simulink model "main_model"  (R2019b)
settings: Solver=FixedStepAuto  StartTime=0.0  StopTime=60.0  FixedStep=0.01  MaxStep=0.01  RelTol=1e-3
values from neighbouring files (symbols this model uses):
  data_array_1 = audioread('Model_Data/Microphone_Data/data_array_1/capture.wav')    [set_workspace_parameters.m]
  data_array_2 = audioread('Model_Data/Microphone_Data/data_array_2/capture.wav')    [set_workspace_parameters.m]
  data_array_3 = audioread('Model_Data/Microphone_Data/data_array_3/capture.wav')    [set_workspace_parameters.m]
undefined symbols (not defined in the file or in its folder): __PRM__SERIALIZED__DATA__, BF, pos, SubsystemReferenceBlock
settings Model: Creator=toons  LastModifiedBy=toons
settings DataIOCC: ExternalInput=[input1, input2]  ReturnWorkspaceOutputs=off
settings DebuggingCC: ArithmeticOperatorsInVariantConditions=warning
settings SFSimCC: CustomCodeUndefinedFunction=UseInterfaceOnly

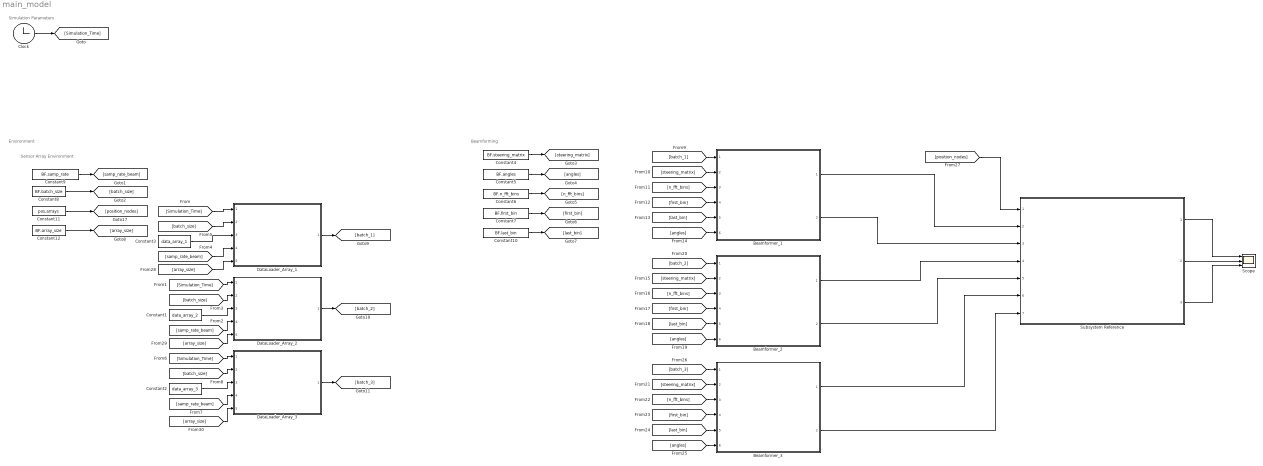
== system main_model ==
  note: Beamforming
  note: Environment
  note: Sensor Array Environment
  note: Simulation Parameters
  Beamformer_1 : Subsystem  BlockKeywords=__PRM__SERIALIZED__DATA__:SubsystemReferenceBlock  ReferencedSubsystem=Beamform_Single_Array
  Beamformer_2 : Subsystem  BlockKeywords=__PRM__SERIALIZED__DATA__:SubsystemReferenceBlock  ReferencedSubsystem=Beamform_Single_Array
  Beamformer_3 : Subsystem  BlockKeywords=__PRM__SERIALIZED__DATA__:SubsystemReferenceBlock  ReferencedSubsystem=Beamform_Single_Array
  Clock : Clock
  Constant1 : Constant  Value=data_array_2  VectorParams1D=off
  Constant10 : Constant  Value=BF.last_bin  VectorParams1D=off
  Constant11 : Constant  Value=pos.arrays  VectorParams1D=off
  Constant12 : Constant  Value=BF.array_size  VectorParams1D=off
  Constant2 : Constant  Value=data_array_3  VectorParams1D=off
  Constant3 : Constant  Value=data_array_1  VectorParams1D=off
  Constant4 : Constant  Value=BF.steering_matrix  VectorParams1D=off
  Constant5 : Constant  Value=BF.angles  VectorParams1D=off
  Constant6 : Constant  Value=BF.n_fft_bins  VectorParams1D=off
  Constant7 : Constant  Value=BF.first_bin  VectorParams1D=off
  Constant8 : Constant  Value=BF.batch_size  VectorParams1D=off
  Constant9 : Constant  Value=BF.samp_rate  VectorParams1D=off
  DataLoader_Array_1 : Subsystem  BlockKeywords=__PRM__SERIALIZED__DATA__:SubsystemReferenceBlock  ReferencedSubsystem=DataLoader_Single_Array
  DataLoader_Array_2 : Subsystem  BlockKeywords=__PRM__SERIALIZED__DATA__:SubsystemReferenceBlock  ReferencedSubsystem=DataLoader_Single_Array
  DataLoader_Array_3 : Subsystem  BlockKeywords=__PRM__SERIALIZED__DATA__:SubsystemReferenceBlock  ReferencedSubsystem=DataLoader_Single_Array
  Scope : Scope  NumInputPorts=3
  Subsystem Reference : Subsystem  BlockKeywords=__PRM__SERIALIZED__DATA__:SubsystemReferenceBlock  ReferencedSubsystem=AnglesToPosition
  wires:
  Clock/1 -> [Simulation_Time]
  Constant3/1 -> DataLoader_Array_1/3
  [Simulation_Time] -> DataLoader_Array_1/1
  Constant9/1 -> [samp_rate_beam]
  [samp_rate_beam] -> DataLoader_Array_1/4
  Constant8/1 -> [batch_size]
  [batch_size] -> DataLoader_Array_1/2
  [batch_size] -> DataLoader_Array_2/2
  Constant1/1 -> DataLoader_Array_2/3
  [Simulation_Time] -> DataLoader_Array_2/1
  [samp_rate_beam] -> DataLoader_Array_2/4
  Constant2/1 -> DataLoader_Array_3/3
  [batch_size] -> DataLoader_Array_3/2
  [samp_rate_beam] -> DataLoader_Array_3/4
  [Simulation_Time] -> DataLoader_Array_3/1
  Constant4/1 -> [steering_matrix]
  Constant5/1 -> [angles]
  Constant6/1 -> [n_fft_bins]
  Constant7/1 -> [first_bin]
  Constant10/1 -> [last_bin]
  DataLoader_Array_1/1 -> [batch_1]
  DataLoader_Array_2/1 -> [batch_2]
  DataLoader_Array_3/1 -> [batch_3]
  [batch_1] -> Beamformer_1/1
  [steering_matrix] -> Beamformer_1/2
  [n_fft_bins] -> Beamformer_1/3
  [first_bin] -> Beamformer_1/4
  [last_bin] -> Beamformer_1/5
  [angles] -> Beamformer_1/6
  [steering_matrix] -> Beamformer_2/2
  [n_fft_bins] -> Beamformer_2/3
  [first_bin] -> Beamformer_2/4
  [last_bin] -> Beamformer_2/5
  [batch_2] -> Beamformer_2/1
  [angles] -> Beamformer_2/6
  [steering_matrix] -> Beamformer_3/2
  [n_fft_bins] -> Beamformer_3/3
  [first_bin] -> Beamformer_3/4
  [last_bin] -> Beamformer_3/5
  [batch_3] -> Beamformer_3/1
  [angles] -> Beamformer_3/6
  Constant11/1 -> [position_nodes]
  [position_nodes] -> Subsystem Reference/1
  Beamformer_1/1 -> Subsystem Reference/2
  Beamformer_1/2 -> Subsystem Reference/3
  Beamformer_2/1 -> Subsystem Reference/4
  Beamformer_2/2 -> Subsystem Reference/5
  Beamformer_3/1 -> Subsystem Reference/6
  Beamformer_3/2 -> Subsystem Reference/7
  Constant12/1 -> [array_size]
  [array_size] -> DataLoader_Array_1/5
  [array_size] -> DataLoader_Array_2/5
  [array_size] -> DataLoader_Array_3/5
  Subsystem Reference/1 -> Scope/1
  Subsystem Reference/2 -> Scope/2
  Subsystem Reference/3 -> Scope/3
